simulink model "motor_von_hw"  (R2026a)
settings: Solver=FixedStepAuto  StopTime=30  FixedStep=0.05  EnableMultiTasking=on
InitFcn:
  | params = load_params();
undefined symbols (not defined in the file or in its folder): dspblkCoreblockFVToolHelper, gcbh
libraries: arduinosensorlib x1, slpidlib x1, arduinolib x1
settings Model: SILPILModeSetting=veronly  ExtModeTrigDuration=2  Creator=j30695fl  LastModifiedBy=j30695fl
settings HardwareCC: ProdBitPerInt=16.0  ProdBitPerPointer=16.0  ProdBitPerSizeT=16.0  ProdBitPerPtrDiffT=16.0  ProdWordSize=8.0  ProdHWDeviceType=Atmel->AVR  UseEmbeddedCoderFeatures=off  UseSimulinkCoderFeatures=off
settings RTWCC: SystemTargetFile=ert.tlc  HardwareBoard=Arduino Uno  TLCOptions=-aInlineSetEventsForThisBaseRateFcn=TLC_FALSE -aSuppressMultiTaskScheduler=TLC_FALSE -aRateBasedStepFcn=1  Toolchain=Arduino AVR  BuildConfiguration=Faster Runs  Description=Embedded Coder
settings ERTTargetCC: ExtModeTransport=3.0  ExtModeAutomaticAllocSize=off  ExtModeStaticAllocSize=250.0  SupportContinuousTime=on  SupportNonInlinedSFcns=on  SupportVariableSizeSignals=on

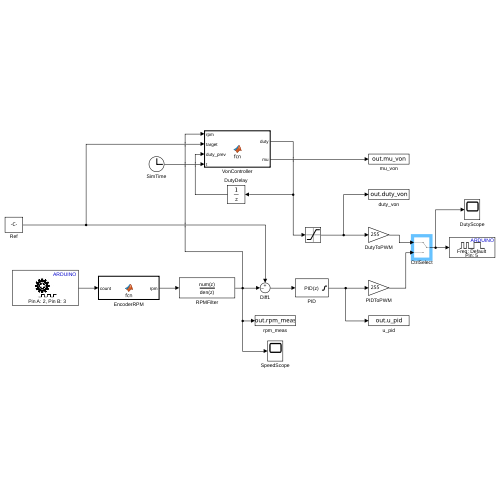
[thumbnail: Simulink's stored preview of the top-level diagram]
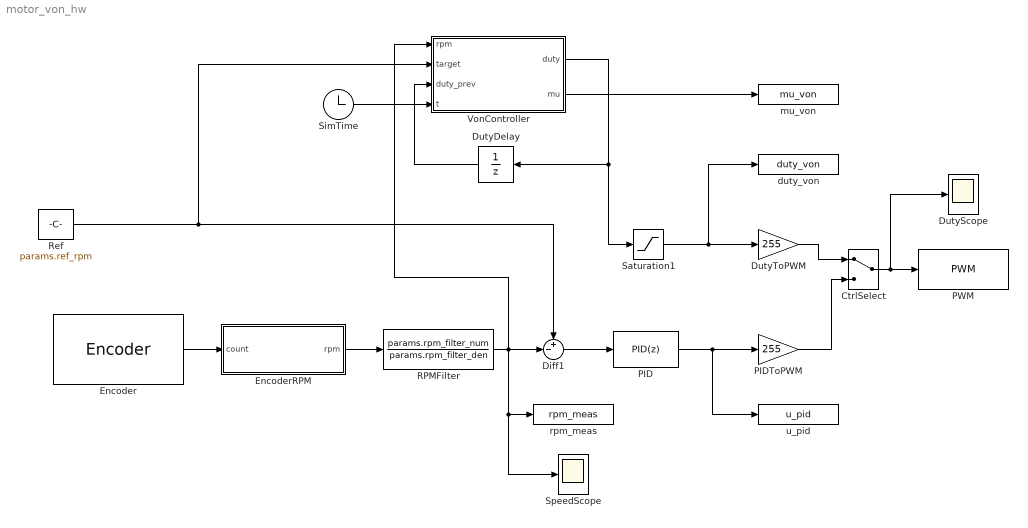
== system motor_von_hw ==
  CtrlSelect : ManualSwitch
  Diff1 : Sum  Inputs=+-|
  DutyDelay : UnitDelay  SampleTime=-1
  DutyScope : Scope
      settings: ActiveDisplayYMinimum=-16.848910680797282  ActiveDisplayYMaximum=200.11896336244723
  DutyToPWM : Gain  Gain=255
  Encoder : arduinosensorlib/Encoder  InputA=2  InputB=3  Mode=No reset  SampleTime=-1
  EncoderRPM : MATLAB Function  TreatAsAtomicUnit=on
  PID : slpidlib/PID Controller  Controller=PID  Form=Parallel  TimeDomain=Discrete-time  UseExternalTs=off  SampleTime=-1  IntegratorMethod=Forward Euler  FilterMethod=Forward Euler  ControllerParametersSource=internal  P=params.pi.kp  I=params.pi.ki  UseKiTs=off  D=0  UseExternalDerivativeSource=off  N=100  UseFilter=on  TunerSelectOption=Transfer Function Based (PID Tuner App)  InitialConditionSource=internal  InitialConditionForIntegrator=0  InitialConditionForFilter=0  DifferentiatorICPrevScaledInput=0  ExternalReset=none  TrackingMode=off  Kt=1  LimitOutput=on  SatLimitsSource=internal  UpperSaturationLimit=1  LowerSaturationLimit=0  LinearizeAsGain=on  AntiWindupMode=clamping  Kb=1  LimitIntegrator=off  UpperIntegratorSaturationLimit=inf  LowerIntegratorSaturationLimit=-inf  POutMin=[]  POutMax=[]  IOutMin=[]  IOutMax=[]  DOutMin=[]  DOutMax=[]  NOutMin=[]  NOutMax=[]  SumOutMin=[]  SumOutMax=[]  SaturationOutMin=[]  SaturationOutMax=[]  PParamMin=[]  PParamMax=[]  IParamMin=[]  IParamMax=[]  DParamMin=[]  DParamMax=[]  NParamMin=[]  NParamMax=[]  KbParamMin=[]  KbParamMax=[]  KtParamMin=[]  KtParamMax=[]  KbOutMin=[]  KbOutMax=[]  KtOutMin=[]  KtOutMax=[]  IntegratorOutMin=[]  IntegratorOutMax=[]  FilterOutMin=[]  FilterOutMax=[]  SumI1OutMin=[]  SumI1OutMax=[]  SumI2OutMin=[]  SumI2OutMax=[]  SumI3OutMin=[]  SumI3OutMax=[]  SumI4OutMin=[]  SumI4OutMax=[]  SumDOutMin=[]  SumDOutMax=[]  DifferentiatorOutMin=[]  DifferentiatorOutMax=[]  FilterDiffOutCoefMin=[]  FilterDiffOutCoefMax=[]  ReciprocalOutMin=[]  ReciprocalOutMax=[]  SumDenOutMin=[]  SumDenOutMax=[]  SumNumOutMin=[]  SumNumOutMax=[]  DivideOutMin=[]  DivideOutMax=[]  UdiffTsProdOutMin=[]  UdiffTsProdOutMax=[]  NTsProdOutMin=[]  NTsProdOutMax=[]  UintegralTsProdOutMin=[]  UintegralTsProdOutMax=[]  UngainTsProdOutMin=[]  UngainTsProdOutMax=[]  ClampingZeroOutDataTypeStr=Inherit: Inherit via back propagation  ClampingZeroOutMin=[]  ClampingZeroOutMax=[]  FilterDenConstantOutDataTypeStr=Inherit: Inherit via back propagation  FilterDenConstantOutMin=[]  FilterDenConstantOutMax=[]  PCopyOutDataTypeStr=Inherit: Inherit via back propagation  PCopyOutMin=[]  PCopyOutMax=[]  NCopyOutDataTypeStr=Inherit: Inherit via back propagation  NCopyOutMin=[]  NCopyOutMax=[]  IntegratorContinuousStateAttributes=''  IntegratorStateMustResolveToSignalObject=off  IntegratorRTWStateStorageClass=Auto  FilterContinuousStateAttributes=''  FilterStateMustResolveToSignalObject=off  FilterRTWStateStorageClass=Auto  ParallelPVariant=InternalParameters  IdealPVariant=Disabled  IVariant=InternalParameters  DVariant=InternalParameters  IntegratorVariant=Discrete  SatVariant=Enabled  AWVariant=DiscClampingParallel  PCopyVariant=Disabled  TRVariant=Disabled  FdbkBlocksVariant=Forward  IdealPFdbkVariant=Disabled  SatFdbkVariant=Disabled  DerivativeFilterVariant=ForwardEulerFilter  NVariant=InternalParameters  NCopyVariant=Disabled  FilterICVariant=InternalICsFilter  IntegratorICVariant=InternalICs  ExternalResetVariant=Disabled  TRSumVariant=Passthrough  SumFdbkVariant=Disabled  SumVariant=Sum_PID  TsampFilterVariant=InternalTs  TsampNgainVariant=Passthrough  TsampIntegralVariant=Disabled_SignalSpec  ExternalSaturationOutDataTypeStr=Inherit: Same as second input  DerivativeSourceVariant=ErrorSignal  PreIntVariant=InternalPreInt
  PIDToPWM : Gain  Gain=255
  PWM : arduinolib/PWM  pinNumber=5  frequencyType=Default  desiredFrequency=490.2  achievableFrequency=490.2
  RPMFilter : DiscreteFilter  LoadFcn=dspblkCoreblockFVToolHelper(gcbh,'load');  Numerator=params.rpm_filter_num  Denominator=params.rpm_filter_den
      settings: CopyFcn=dspblkCoreblockFVToolHelper(gcbh,'copy');  DeleteFcn=dspblkCoreblockFVToolHelper(gcbh,'close');  ModelCloseFcn=dspblkCoreblockFVToolHelper(gcbh,'close');  PreSaveFcn=dspblkCoreblockFVToolHelper(gcbh,'presave');  PostSaveFcn=dspblkCoreblockFVToolHelper(gcbh,'postsave');  CloseFcn=dspblkCoreblockFVToolHelper(gcbh,'close');
  Ref : Constant  Value=params.ref_rpm
  Saturation1 : Saturate  UpperLimit=1  LowerLimit=0
  SimTime : Clock
  SpeedScope : Scope
      settings: ActiveDisplayYMinimum=-4.8874729265852546  ActiveDisplayYMaximum=43.9872563392673
  VonController : MATLAB Function  TreatAsAtomicUnit=on
  duty_von : ToWorkspace  VariableName=duty_von  SaveFormat=Timeseries  SampleTime=-1
  mu_von : ToWorkspace  VariableName=mu_von  SaveFormat=Timeseries  SampleTime=-1
  rpm_meas : ToWorkspace  VariableName=rpm_meas  SaveFormat=Timeseries  SampleTime=-1
  u_pid : ToWorkspace  VariableName=u_pid  SaveFormat=Timeseries  SampleTime=-1
  wires:
  Ref/1 -> Diff1/1, VonController/2(target)
  RPMFilter/1 -> VonController/1(rpm), SpeedScope/1, rpm_meas/1, Diff1/2
  DutyToPWM/1 -> CtrlSelect/1
  PIDToPWM/1 -> CtrlSelect/2
  CtrlSelect/1 -> DutyScope/1, PWM/1
  PID/1 -> u_pid/1, PIDToPWM/1
  Diff1/1 -> PID/1
  DutyDelay/1 -> VonController/3(duty_prev)
  VonController/1(duty) -> Saturation1/1, DutyDelay/1
  VonController/2(mu) -> mu_von/1
  Saturation1/1 -> duty_von/1, DutyToPWM/1
  Encoder/1 -> EncoderRPM/1(count)
  EncoderRPM/1(rpm) -> RPMFilter/1
  SimTime/1 -> VonController/4(t)

== matlab function motor_von_hw/EncoderRPM ==
  data: count input; rpm output
function rpm = fcn(count)
coder.extrinsic('encoder_rpm');
rpm = 0;
rpm = encoder_rpm(count);
end

== matlab function motor_von_hw/VonController ==
  settings: updateMethod=DISCRETE
  data: rpm input; duty output; target input; duty_prev input; mu output; t input
function [duty, mu] = fcn(rpm, target, duty_prev, t)
coder.extrinsic('von_fuzzy');
duty = 0; mu = zeros(9,1);
[duty, mu] = von_fuzzy(rpm, target, duty_prev, t);
end
